simulink model "excercise1_3bd2"  (R2024b)
settings: Solver=ode45  StartTime=0.0  StopTime=3  MaxStep=0.001  RelTol=1e-3
undefined symbols (not defined in the file): d, k, m
settings Model: Creator=elliot  LastModifiedBy=elliot
settings RTWCC: GPUComputeCapability=3.5

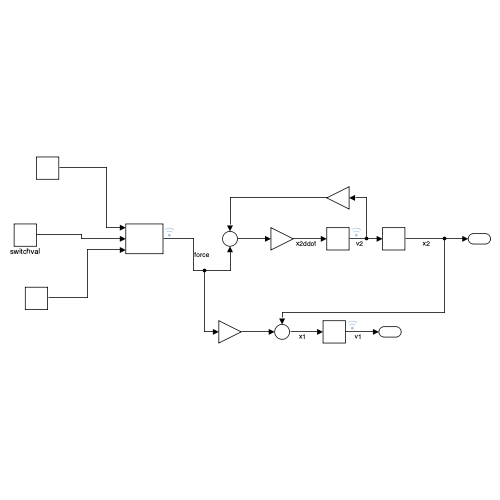
[thumbnail: Simulink's stored preview of the top-level diagram]
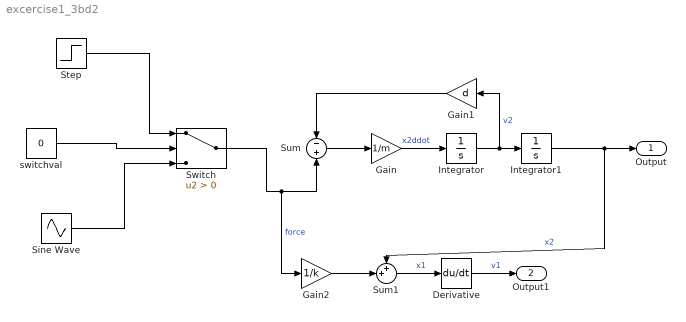
== system excercise1_3bd2 ==
  Derivative : Derivative
  Gain : Gain  Gain=1/m
  Gain1 : Gain  Gain=d
  Gain2 : Gain  Gain=1/k
  Integrator : Integrator
  Integrator1 : Integrator
  Sine Wave : Sin  Frequency=200  SampleTime=0
  Step : Step  SampleTime=0
  Sum : Sum  Inputs=-+
  Sum1 : Sum  Inputs=++|
  Switch : Switch  Criteria=u2 > Threshold  SaturateOnIntegerOverflow=off  InputSameDT=off
  switchval : Constant  Value=0
  Output : Outport
  Output1 : Outport  Port=2
  wires:
  Sum/1 -> Gain/1
  switchval/1 -> Switch/2
  Step/1 -> Switch/1
  Switch/1 -> Gain2/1, Sum/2  "force"
  Sine Wave/1 -> Switch/3
  Gain/1 -> Integrator/1  "x2ddot"
  Integrator/1 -> Gain1/1, Integrator1/1  "v2"
  Gain1/1 -> Sum/1
  Integrator1/1 -> Sum1/1, Output/1  "x2"
  Gain2/1 -> Sum1/2
  Sum1/1 -> Derivative/1  "x1"
  Derivative/1 -> Output1/1  "v1"
